simulink model "TVCRocketSimulation_REV_0"  (R2021a)
settings: Solver=VariableStepAuto  StartTime=0.0  StopTime=10.0  RelTol=1e-3
libraries: simulink x2, simulink_extras x1, shared3dof x1
settings Model: Creator=ian  LastModifiedBy=elija

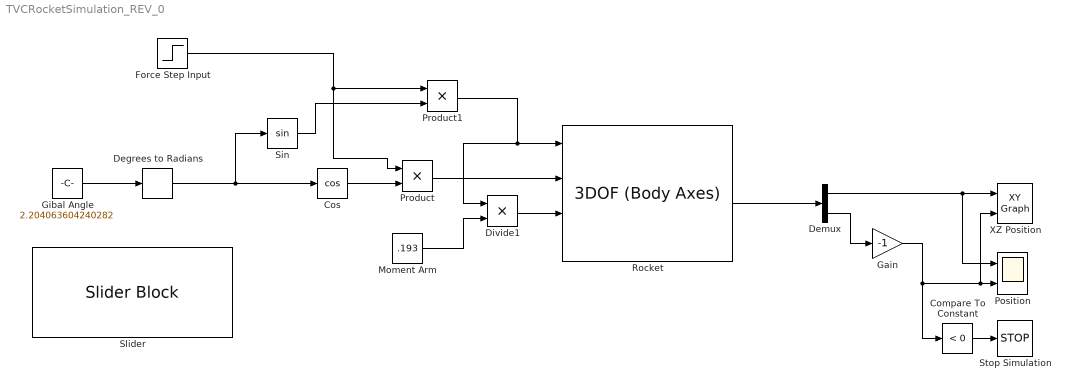
== system TVCRocketSimulation_REV_0 ==
  Compare To Constant : simulink/Logic and Bit Operations/Compare To Constant  relop=<  const=0  OutDataTypeStr=boolean
  Cos : Trigonometry  Operator=cos
  Degrees to Radians : simulink_extras/Transformations/Degrees to Radians
  Demux : Demux  Outputs=2
  Divide1 : Product  Inputs=**
  Force Step Input : Step  Time=2.4  Before=-15  After=0  SampleTime=0
  Gain : Gain  Gain=-1
  Gibal Angle : Constant  Value=2.204063604240282
  Moment Arm : Constant  Value=.193
  Position : Scope  NumInputPorts=2
  Product : Product  RndMeth=Zero
  Product1 : Product  RndMeth=Zero
  Rocket : shared3dof/3DOF (Body Axes)  units=Metric (MKS)  mtype=Fixed  v_ini=0  theta_ini=0  alpha_ini=0  pos_ini=[0 0]  q_ini=0  mass=.805  mass_e=0.5  mass_f=3.0  Iyy=.017  Iyy_e=0.5  Iyy_f=3.0  g_in=External  g=9.81  vre_flag=on  abi_flag=off  aMode=0  vel_statename=''  theta_statename=''  pos_statename=''  q_statename=''  mass_statename=''
      settings: SourceProductBaseCode=AE,PW,DR,MT,UV,VE
  Sin : Trigonometry
  Slider : SliderBlock  ScaleMin=-5  ScaleMax=5
  Stop Simulation : Stop
  XZ Position : simulink/Sinks/XY Graph  xmin=-20  xmax=20  ymin=0  ymax=20  st=-1
  wires:
  Rocket/4 -> Demux/1
  Demux/1 -> Position/1, XZ Position/1
  Compare To Constant/1 -> Stop Simulation/1
  Force Step Input/1 -> Product1/1, Product/1
  Gibal Angle/1 -> Degrees to Radians/1
  Cos/1 -> Product/2
  Product1/1 -> Rocket/1, Divide1/1
  Sin/1 -> Product1/2
  Product/1 -> Rocket/2
  Moment Arm/1 -> Divide1/2
  Degrees to Radians/1 -> Cos/1, Sin/1
  Demux/2 -> Gain/1
  Gain/1 -> XZ Position/2, Position/2, Compare To Constant/1
  Divide1/1 -> Rocket/3
